simulink model "HPF_Activity2"  (R2022a)
settings: Solver=VariableStepAuto  StartTime=0.0  StopTime=10.0  FixedStep=.000000001  RelTol=1e-3
libraries: dspfdesign x2, dspsrcs4 x1
settings Model: Creator=chadw  LastModifiedBy=chadw

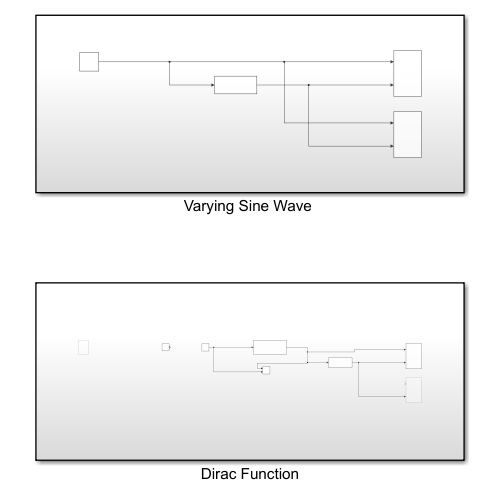
[thumbnail: Simulink's stored preview of the top-level diagram]
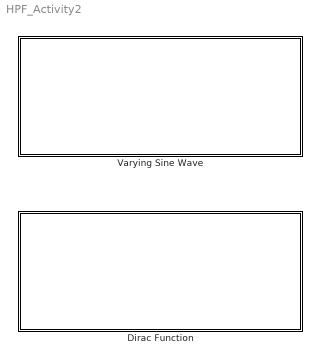
== system HPF_Activity2 ==
  Dirac Function : Subsystem
  "Varying Sine Wave " : Subsystem

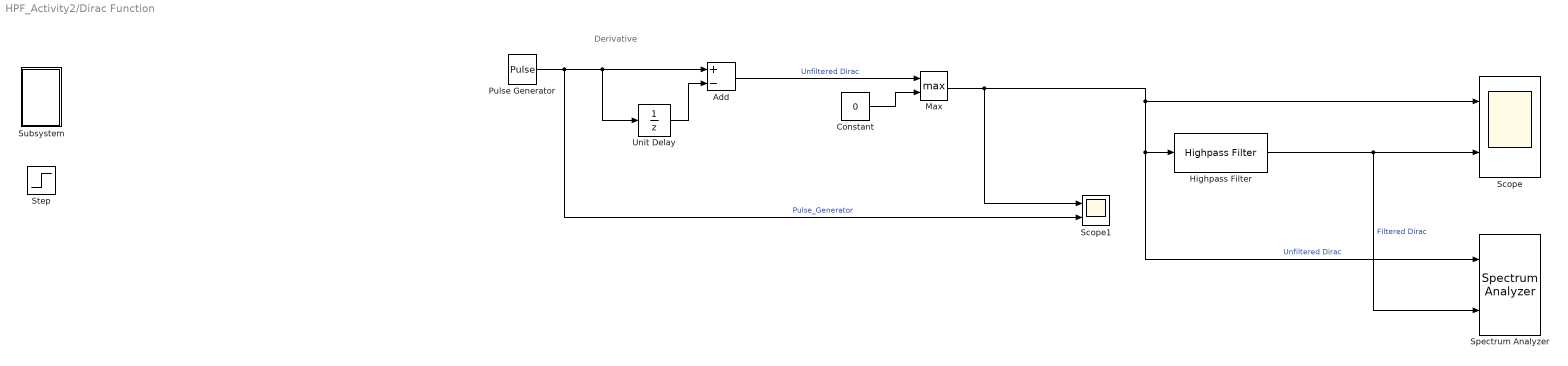
== system HPF_Activity2/Dirac Function ==
  note: Derivative
  Add : Sum  Inputs=+-
  Constant : Constant  Value=0
  Highpass Filter : dspfdesign/Highpass Filter  FilterType=FIR  DesignForMinimumOrder=on  FilterOrder=50  StopbandFrequency=HPF_StopBand_Freq  PassbandFrequency=HPF_PassBand_Freq  StopbandAttenuation=HPF_StopBand_Amp  PassbandRipple=HPF_PassBand_Amp  InheritSampleRate=off  SampleRate=44100  SimulateUsing=Interpreted execution  roundingMode=Floor  coeffsDataTypeStr=fixdt(1,16)
  Max : MinMax  Function=max  Inputs=2
  Pulse Generator : DiscretePulseGenerator  Period=2000  PulseWidth=5  PhaseDelay=10  SampleTime=1/1000
  Scope : Scope  NumInputPorts=2
  Scope1 : Scope  NumInputPorts=2
  Spectrum Analyzer : SpectrumAnalyzer  NumInputPorts=2
  Step : Step  SampleTime=1/1000
  Subsystem : Subsystem
  Unit Delay : UnitDelay  SampleTime=-1  HasFrameUpgradeWarning=on
  wires:
  Highpass Filter/1 -> Spectrum Analyzer/2, Scope/2  "Filtered Dirac"
  Pulse Generator/1 -> Scope1/2, Unit Delay/1, Add/1  "Pulse_Generator"
  Max/1 -> Spectrum Analyzer/1, Highpass Filter/1, Scope/1, Scope1/1  "Unfiltered Dirac"
  Constant/1 -> Max/2
  Unit Delay/1 -> Add/2
  Add/1 -> Max/1  "Unfiltered Dirac"

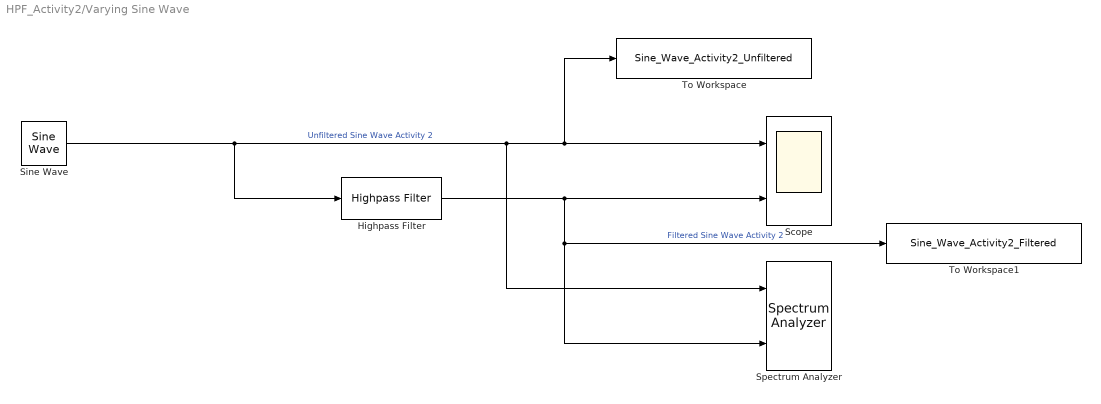
== system HPF_Activity2/Varying Sine Wave  ==
  Highpass Filter : dspfdesign/Highpass Filter  FilterType=FIR  DesignForMinimumOrder=on  FilterOrder=50  StopbandFrequency=HPF_StopBand_Freq  PassbandFrequency=HPF_PassBand_Freq  StopbandAttenuation=HPF_StopBand_Amp  PassbandRipple=HPF_PassBand_Amp  InheritSampleRate=off  SampleRate=44100  SimulateUsing=Interpreted execution  roundingMode=Floor  coeffsDataTypeStr=fixdt(1,16)
  Scope : Scope  NumInputPorts=2
  Sine Wave : dspsrcs4/Sine Wave  Amplitude=1  Frequency=[10, 100, 200, 400]  Phase=0  SampleMode=Discrete  OutComplex=Real  CompMethod=Trigonometric fcn  TableSize=Speed  SampleTime=1/1000  SamplesPerFrame=1  ResetState=Restart at time zero  OutputFrames=off  dataType=double  wordLen=16  udDataType=sfix(16)  fracBitsMode=Best precision  numFracBits=15  OutDataTypeStr=double  LastOutDataTypeStr=double
  Spectrum Analyzer : SpectrumAnalyzer  NumInputPorts=2
  To Workspace : ToWorkspace  VariableName=Sine_Wave_Activity2_Unfiltered  SaveFormat=Timeseries  SampleTime=-1
  To Workspace1 : ToWorkspace  VariableName=Sine_Wave_Activity2_Filtered  SaveFormat=Timeseries  SampleTime=-1
  wires:
  Highpass Filter/1 -> Scope/2, Spectrum Analyzer/2, To Workspace1/1  "Filtered Sine Wave Activity 2"
  Sine Wave/1 -> Highpass Filter/1, To Workspace/1, Scope/1, Spectrum Analyzer/1  "Unfiltered Sine Wave Activity 2"

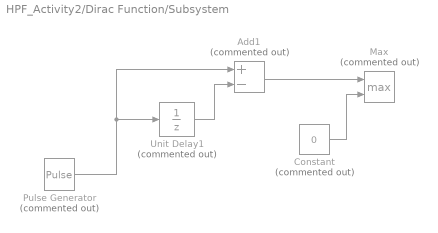
== system HPF_Activity2/Dirac Function/Subsystem ==
  Add1 : Sum  Commented=on  Inputs=+-
  Constant : Constant  Commented=on  Value=0
  Max : MinMax  Commented=on  Function=max  Inputs=2
  Pulse Generator : DiscretePulseGenerator  Commented=on  PulseType=Time based  Period=10  PulseWidth=5  PhaseDelay=2
  Unit Delay1 : UnitDelay  Commented=on  SampleTime=-1  HasFrameUpgradeWarning=on
  wires:
  Unit Delay1/1 -> Add1/2
  Pulse Generator/1 -> Unit Delay1/1, Add1/1
  Add1/1 -> Max/1
  Constant/1 -> Max/2
